simulink model "planta_no_lineal"  (R2023b)
settings: Solver=ode45  StartTime=0.0  StopTime=14400  MaxStep=0.01  RelTol=1e-3
model workspace (MAT data in the model file):
  max = 0.5
  min = 0
libraries: simulink x1
settings Model: Creator=q  LastModifiedBy=q

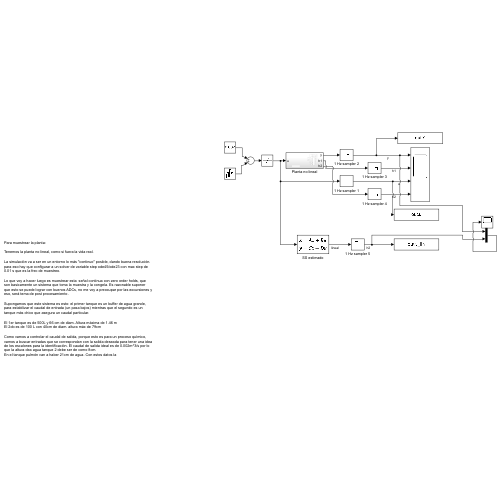
[thumbnail: Simulink's stored preview of the top-level diagram]
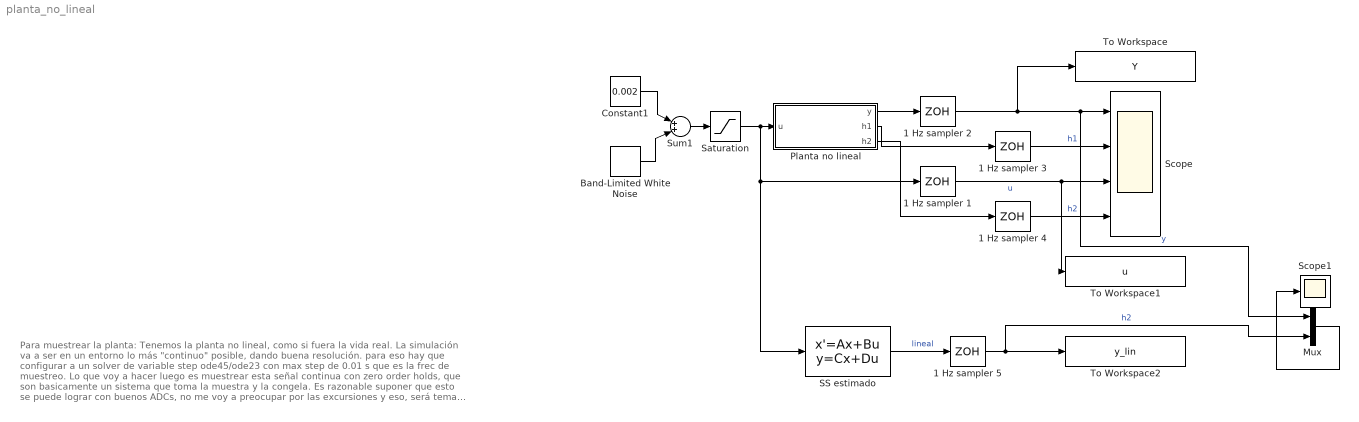
== system planta_no_lineal ==
  note: Para muestrear la planta:
      |
      | Tenemos la planta no lineal, como si fuera la vida real.
      |
      | La simulación va a ser en un entorno lo más "continuo" posible, dando buena resolución. para eso hay que configurar a un solver de variable step ode45/ode23 con max step de 0.01 s que es la frec de muestreo.
      |
      | Lo que voy a hacer luego es muestrear esta  señal continua con zero order holds, que son basicamente un sistema que toma la muestra y la congela. Es razonable suponer que esto se puede lograr con buenos ADCs, no me voy a preocupar por las excursiones y eso, será tema de post procesamiento .
      |
      | Supongamos que este sistema es esto: el primer tanque es un buffer de agua grande, para estabilizar el caudal de entrada (un pasa bajos) mientras que el segundo es un tanque más chico que asegura un caudal particular.
      |
      | El 1er tanque es de 500L y 66 cm de diam. Altura máxima de 1.46 m
      | El 2do es de 100 L con 40cm de diam. altura máx de 79cm
      |
      | Como vamos a controlar el caudal de salida, porque esto es para un proceso químico, vamos a buscar entradas que se correspondan con la salida deseada para tener una idea de los escalones para la identificación. El caudal de salida ideal es de 0.002m^3/s por lo que la altura dea agua tanque 2 debe ser de como 8cm.
      | En el tanque pulmón van a haber 21cm de agua. Con estos datos la
  1 Hz sampler {1..5} (5 alike) : ZeroOrderHold
  Band-Limited White Noise : simulink/Sources/Band-Limited White Noise  Cov=[0.000002]  Ts=200  seed=[23341]
  Constant1 : Constant  Value=0.002
  Mux : Mux  Inputs=2
  Planta no lineal : Subsystem
  SS estimado : StateSpace  A=[-0.023375234759513,0.035713459182280;0.016442055191371,-0.031577082096728]  B=[2.537448139699421;-1.771387482474186]  C=[0.008723840649702,0.012539591066566]  D=0  InitialCondition=0
  Saturation : Saturate  UpperLimit=0.0022  LowerLimit=0.0018
  Scope : Scope  NumInputPorts=4
  Scope1 : Scope
  Sum1 : Sum  Inputs=|++|
  To Workspace : ToWorkspace  VariableName=Y  SampleTime=1
  To Workspace1 : ToWorkspace  VariableName=u  SampleTime=1
  To Workspace2 : ToWorkspace  VariableName=y_lin  SampleTime=1
  wires:
  Planta no lineal/1(y) -> 1 Hz sampler 2/1
  1 Hz sampler 2/1 -> To Workspace/1, Mux/1, Scope/1  "y"
  1 Hz sampler 1/1 -> To Workspace1/1, Scope/3  "u"
  Planta no lineal/2(h1) -> 1 Hz sampler 3/1
  Planta no lineal/3(h2) -> 1 Hz sampler 4/1
  1 Hz sampler 3/1 -> Scope/2  "h1"
  1 Hz sampler 4/1 -> Scope/4  "h2"
  Constant1/1 -> Sum1/1
  Band-Limited White Noise/1 -> Sum1/2
  Sum1/1 -> Saturation/1
  Saturation/1 -> SS estimado/1, 1 Hz sampler 1/1, Planta no lineal/1(u)
  SS estimado/1 -> 1 Hz sampler 5/1  "lineal"
  1 Hz sampler 5/1 -> Mux/2, To Workspace2/1  "h2"
  Mux/1 -> Scope1/1

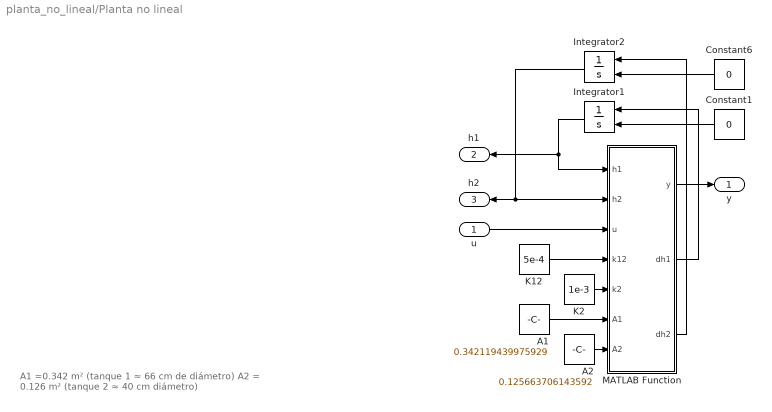
== system planta_no_lineal/Planta no lineal ==
  note: A1 =0.342   m²   (tanque 1 ≈ 66 cm de diámetro)
      | A2 = 0.126   m²   (tanque 2 ≈ 40 cm diámetro)
  u : Inport
  A1 : Constant  Value=0.342119439975929
  A2 : Constant  Value=0.125663706143592
  Constant1 : Constant  Value=0
  Constant6 : Constant  Value=0
  Integrator1 : Integrator  InitialConditionSource=external
  Integrator2 : Integrator  InitialConditionSource=external
  K12 : Constant  Value=5e-4
  K2 : Constant  Value=1e-3
  MATLAB Function : MATLAB Function  TreatAsAtomicUnit=on
  y : Outport
  h1 : Outport  Port=2
  h2 : Outport  Port=3
  wires:
  Integrator2/1 -> h2/1, MATLAB Function/2(h2)
  MATLAB Function/2(dh1) -> Integrator1/1
  K2/1 -> MATLAB Function/5(k2)
  Integrator1/1 -> h1/1, MATLAB Function/1(h1)
  Constant1/1 -> Integrator1/2
  A2/1 -> MATLAB Function/7(A2)
  MATLAB Function/3(dh2) -> Integrator2/1
  MATLAB Function/1(y) -> y/1
  Constant6/1 -> Integrator2/2
  K12/1 -> MATLAB Function/4(k12)
  A1/1 -> MATLAB Function/6(A1)
  u/1 -> MATLAB Function/3(u)

== matlab function planta_no_lineal/Planta no lineal/MATLAB Function ==
  data: h1 input; h2 input; y output; dh1 output; u input; k12 input; k2 input; A1 input; A2 input; dh2 output
function [y, dh1, dh2] = fcn(h1, h2, u, k12, k2, A1, A2)
g = 9.81;

delta_h = max(h1 - h2, 0);

q12 = k12 * sqrt(2 * g * delta_h); % caudal intermedio
q2  = k2  * sqrt(2 * g * max(h2, 0)); % caudal de salida

dh1 = (u - q12) / A1;
dh2 = (q12 - q2) / A2;

y = q2;

%el modelo asume flujo solo en un sentido

%se ignora inversión de flujo

%el sistema es válido para niveles positivos
